simulink model "Mass_Springs_Systems"  (R2021b)
settings: Solver=ode4  StartTime=0.0  StopTime=30  FixedStep=.001  RelTol=1e-3  AbsTol=1e-3  EnableMultiTasking=on
model workspace (MAT data in the model file):
  cslide = 0.25
  iz = [0.192  0.091; 0.207  0.094; 0.221  0.104; 0.238  0.118; 0.251  0.141; 0.262  0.168; 0.268  0.205; 0.27  0.242; 0.267  0.277; 0.262  0.308; 0.246  0.348; 0.232  0.369; 0.206  0.39; 0.185  0.39; 0.16  0.377; 0.137  0.349; 0.126  0.325; 0.118  0.297; 0.114  0.265; 0.113  0.237; 0.118  0.191; 0.128  0.156; 0.139  0.13; 0.156  0.107; 0.175  0.096]
  m1 = 0
  m2 = 0
  m3 = 0
  one = [0.064  0.072; 0.088  0.03; 0.169  0.03; 0.168  0.458; 0.129  0.458; 0.128  0.073]
  smiData.RigidTransform.translation = [-21.5561986301 -14.8674859839 15.0728144895]
  smiData.RigidTransform.angle = 0
  smiData.RigidTransform.axis = [0 0 0]
  smiData.RigidTransform.ID = 'RootGround[rack-1]'
  smiData.Solid.mass = 0.0200061588425
  smiData.Solid.CoM = [0 0.838779102261 -0.00603396973069]
  smiData.Solid.MoI = [0.670200057653 0.669872690066 0.00366172739385]
  smiData.Solid.PoI = [5.56695055283e-05 0 0]
  smiData.Solid.color = [0.792156862745 0.819607843137 0.933333333333]
  smiData.Solid.opacity = 1
  smiData.Solid.ID = 'rack*:*Default'
  three = [0.252  0.12; 0.239  0.091; 0.214  0.068; 0.179  0.053; 0.14  0.052; 0.107  0.064; 0.083  0.082; 0.065  0.121; 0.075  0.155; 0.102  0.176; 0.129  0.188; 0.163  0.194; 0.182  0.194; 0.183  0.24; 0.131  0.247; 0.099  0.256; 0.068  0.28; 0.048  0.313; 0.047  0.345; 0.055  0.378; 0.084  0.41; 0.127  0.429; 0.179  0.43; 0.214  0.419; 0.246  0.396; 0.26  0.368; 0.269  0.344; 0.311  0.344; 0.303  0.374; 0.29  0.409; 0.262  0.442; 0.23  0.463; 0.18  0.475; 0.137  0.476; 0.097  0.465; 0.057  0.441; 0.028  0.411; 0.011  0.374; 0.006  0.353; 0.01  0.295; 0.028  0.258; 0.05  0.233; 0.08  0.214; 0.06  0.196; 0.041  0.175; 0.029  0.135; 0.029  0.104; 0.043  0.066; 0.074  0.032; 0.106  0.015; 0.147  0.006; 0.187  0.007; 0.223  0.021; 0.255  0.044; 0.278  0.081; 0.294  0.119]
  two = [0.081  0.154; 0.042  0.154; 0.05  0.108; 0.06  0.085; 0.082  0.055; 0.106  0.033; 0.135  0.02; 0.161  0.013; 0.194  0.014; 0.226  0.02; 0.253  0.032; 0.279  0.054; 0.297  0.083; 0.305  0.109; 0.309  0.141; 0.306  0.168; 0.299  0.189; 0.281  0.221; 0.242  0.271; 0.119  0.401; 0.315  0.403; 0.314  0.445; 0.027  0.446; 0.242  0.214; 0.263  0.177; 0.272  0.145; 0.264  0.106; 0.243  0.079; 0.208  0.059; 0.185  0.058; 0.162  0.06; 0.133  0.067; 0.12  0.076; 0.102  0.092; 0.088  0.119; 0.085  0.134]
  xy_simple = [39.1661  19.7032018238; 3.8339  19.7032; -0.28263658  19.7032; -0.28263658  0; 43  0; 43  19.7032]
  zero = [0.2  0.026; 0.245  0.033; 0.288  0.063; 0.316  0.099; 0.335  0.149; 0.345  0.197; 0.347  0.246; 0.344  0.292; 0.338  0.339; 0.324  0.384; 0.3  0.429; 0.269  0.456; 0.223  0.475; 0.173  0.475; 0.132  0.46; 0.097  0.426; 0.072  0.383; 0.062  0.338; 0.058  0.289; 0.058  0.242; 0.059  0.192; 0.068  0.145; 0.083  0.102; 0.111  0.062; 0.149  0.037]
undefined symbols (not defined in the file): A, d1, d2, ha, X, Y, Z
libraries: sm_lib x6312, nesl_utility x38
(part 1 of 121)
settings Model: Creator=HP Owner  LastModifiedBy=acontr14
settings SolverCC: AutoScaleAbsTol=off  AlgebraicLoopSolver=TrustRegion
settings DataIOCC: MaxDataPoints=10000
settings OptimizationCC: LifeSpan=inf
settings DebuggingCC: AllowSymbolicDim=off  SFUnexpectedBacktrackingDiag=warning  SFNoUnconditionalDefaultTransitionDiag=warning  SFExecutionAtInitializationDiag=none  SFMachineParentedDataDiag=warning  ArithmeticOperatorsInVariantConditions=warning
settings SFSimCC: SimUseLocalCustomCode=off  CustomCodeUndefinedFunction=UseInterfaceOnly
settings RTWCC: RTWUseLocalCustomCode=off
settings CodeAppCC: StateflowObjectComments=on
settings GRTTargetCC: TargetLangStandard=C89/C90 (ANSI)
settings ConfigComp: CovMetricSettings=dw  CovSaveCumulativeToWorkspaceVar=on  CovSaveSingleToWorkspaceVar=on  CovExternalEMLEnable=off  CovSFcnEnable=off
settings SimscapeCC: SimscapeLogType=all  SimscapeLogSimulationStatistics=on  SimscapeLogDataHistory=10000

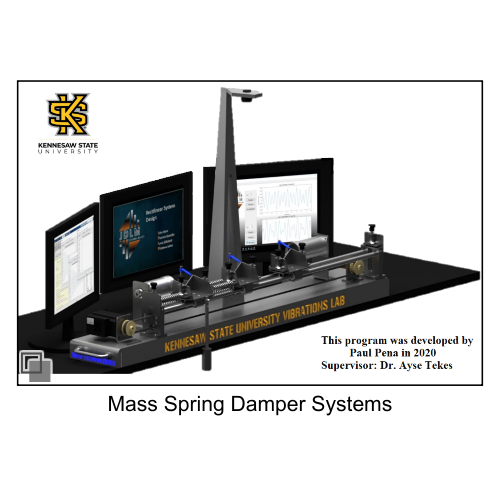
[thumbnail: Simulink's stored preview of the top-level diagram]
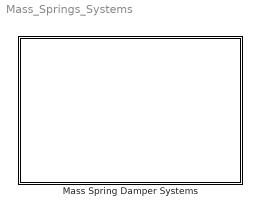
== system Mass_Springs_Systems ==
  Mass Spring Damper Systems : Subsystem  Variant=on  VariantControlMode=label  VariantControl=MS  LabelModeActiveChoice=22ms
      mask Display: image('$imagefile'); % Use "Edit Image" on toolstrip to change.

== system Mass_Springs_Systems/Mass Spring Damper Systems ==
  note: 1 Mass 1 Spring
  note: 3 Mass 3 Spring
  note: 2 Mass 2 Spring
  note: 1 Mass 2 Spring
  note: 2 Mass 3 Spring
  2Masses 2Springs : Subsystem  AncestorBlock=Lib/2Masses 2Springs  VariantControl=22ms  mask{m1=2, m2=1, k1=600, k2=400, d=1, s_f=.35, id1=2, id2=2, zero_forces=on, zerodis=off, force_type=Harmonic, Force=1, Har_Force=1, freq=sqrt(400/1.5)}
      mask prompts: m1 "Mass1 (kg)"; m2 "Mass2 (kg)"; k1 "K1 Spring Constant (N/m)"; k2 "K2 Spring Constant (N/m)"; d "Spring Damping (kg/s)"; s_f "Surface Friction (N/(m/s))"; id1 "M1 Initial Displacement (cm)"; id2 "M2 Initial Displacement (cm)"; zero_forces "Zero Forces"; zerodis "Zero Initial Displacement"; force_type "Force Response Type"; Force "Magnitude(N)"; Har_Force "Magnitude(N)"; freq "Frequency(rad/s)"
      mask init:
      | switch force_type
      |     case 1
      |         Har_Force = 0;
      |         freq = 0;
      |     case 2
      |         Force = 0;
      | end
      | if zero_forces == 1
      |     Har_Force = 0;
      |     Force = 0;
      |     freq = 0;
      | end
      | 
      | if zerodis == 1
      |     id1=0;
      |     id2=0;
      | end
      mask Callback zero_forces:
      | % Enable and disable parameters
      | 
      | % Get the value of the Enable Bias checkbox
      | % unchecked = 'off'
      | % checked = 'on'
      | enab = get_param(gcb,'zero_forces');
      | 
      | % Set the 'MaskEnables' property for each parameters
      | if strcmp(enab,'on')
      |     set_param(gcb,'MaskVisibilities',{'on','on','on','on','on','on','on','on','on','off','off','off','off','off'});
      | else
      |     set_param(gcb,'MaskVisibilities',{'on','on','on','on','on','on','on','on','on','on','on','on','on','on'});
      | end
      | 
      | % Note that the value of the bias is not handled here.
      | % See the Initialization tab
      mask Callback zerodis:
      | % Enable and disable parameters
      | 
      | % Get the value of the Enable Bias checkbox
      | % unchecked = 'off'
      | % checked = 'on'
      | enab = get_param(gcb,'zerodis');
      | 
      | % Set the 'MaskEnables' property for each parameters
      | if strcmp(enab,'on')
      |     set_param(gcb,'MaskEnables',{'on','on','on','on','on','on','off','off','on','on','on','on','on','on'});
      | else
      |     set_param(gcb,'MaskEnables',{'on','on','on','on','on','on','on','on','on','on','on','on','on','on'});
      | end
      | 
      | % Note that the value of the bias is not handled here.
      | % See the Initialization tab
      mask TypeOptions force_type: Step | Harmonic
      mask DialogControl Control4 Prompt: Update Model
      mask DialogControl Control4 Callback: set_param(bdroot,'SimulationCommand','update')
      mask DialogControl Control2 Prompt: Run Simulation
      mask DialogControl Control2 Callback: set_param(bdroot,'SimulationCommand','start')
      mask DialogControl Control3 Prompt: STOP Simulation
      mask DialogControl Control3 Callback: set_param(bdroot,'SimulationCommand','stop')
      mask DialogControl Control7 Prompt: Open Scope Plot
      mask DialogControl Control7 Callback: open(Simulink.BlockPath({'Mass_Springs_Systems/Mass Spring Damper Systems/2Masses 2Springs/Position'}))
      mask DialogControl Control14 Prompt: Frequency Plot
      mask DialogControl Control14 Callback:
      | cart1=evalin('base','out.pos1');
      | cart2=evalin('base','out.pos2');
      | time=evalin('base','out.tout');
      | 
      | Ts = time(2)-time(1);
      | fs = 1/Ts;
      | N = length(cart1);
      | 
      | Y1 = abs(fft(cart1)/N); % fft of cart1 data
      | Y1d = Y1(1:N/2+1); %single side spectrum
      | Y1d(2:end-1) = 2*Y1d(2:end-1); %amplitude adjustment
      | 
      | Y2 = abs(fft(cart2)/N);
      | Y2d = Y2(1:N/2+1);
      | Y2d(2:end-1) = 2*Y2d(2:end-1);
      | 
      | 
      | f = fs*(0:(N/2))/N; %create frequency vector
      | 
      | figure;
      | plot(f,Y1d); xlim([0 10]);
      | hold on;
      | plot(f,Y2d,'r')
      | hold off;
      mask DialogControl Control16 Prompt: Mode Ratios
      mask DialogControl Control16 Callback:
      | syms  w
      | m1=get_param(gcb,'m1');
      | m1=str2double(m1);
      | m2=get_param(gcb,'m2');
      | m2=str2double(m2);
      | k1=get_param(gcb,'k1');
      | k1=str2double(k1);
      | k2=get_param(gcb,'k2');
      | k2=str2double(k2);
      | M=[k1+k2-m1*w^2 -k2; -k2 k2-m2*w^2];
      | detM=det(M);
      | solution=double(solve(detM==0,w));
      | pos=solution>0;
      | wsolution=solution(pos);
      | w1=wsolution(1);
      | w2=wsolution(2);
      | f1=w1/(2*pi);
      | f2=w2/(2*pi);
      | M1=double(subs(M,w,w1));
      | Mode_Ratio_1=M1(1,1)/-M1(1,2);
      | M2=double(subs(M,w,w2));
      | Mode_Ratio_2=M2(1,1)/-M2(1,2);
      | %set_param(gcb,'MaskSelfModifiable','on');
      | % Get the mask object
      | mo = get_param(gcb,'MaskObject');
      | % Get the text object
      | tc = mo.getDialogControl('TextControl1');
      | % Change the string
      | tc.Prompt = string(Mode_Ratio_1);
      | % Get the text object
      | tc = mo.getDialogControl('TextControl2');
      | % Change the string
      | tc.Prompt = string(Mode_Ratio_2);
      mask DialogControl Container6 Prompt: Variables
      mask DialogControl Control13 Prompt: (Add text here)
      mask DialogControl Container8 Prompt: Free Response
      mask DialogControl Container11 Prompt: Free Response
      mask DialogControl Control17 Prompt: Mode Ratio of Mass 1:
      mask DialogControl TextControl1 Prompt: 1.6861
      mask DialogControl Control19 Prompt: Mode Ratio of Mass 2:
      mask DialogControl TextControl2 Prompt: -1.1861
      mask DialogControl Control10 Prompt: "Check Box below for Only Free Response"
      mask DialogControl Container19 Prompt: Forced Response
      mask DialogControl Container10 Prompt: Forced Response
      mask DialogControl Control9 Prompt: Uncheck "Zero Forces" in Free Response Tab to add Forced Response
      mask DialogControl Container13 Prompt: Step Response
      mask DialogControl Container16 Prompt: Harmonic Response
      mask Display: image('$imagefile'); % Use "Edit Image" on toolstrip to change.
  2Masses 3Springs : Subsystem  AncestorBlock=Lib/2Masses 3Springs  VariantControl=23ms  mask{m1=2, m2=2, k1=700, k2=300, k3=700, d=1/3, s_f=0, id1=3.500, id2=-3.500, zero_forces=on, zerodis=off, force_type=Harmonic, Force=5, Har_Force=3, freq=20}
      mask prompts: m1 "Mass1 (kg)"; m2 "Mass2 (kg)"; k1 "K1 Spring Constant (N/m)"; k2 "K2 Spring Constant (N/m)"; k3 "K3 Spring Constant (N/m)"; d "Spring Damping (kg/s)"; s_f "Surface Friction (N/(m/s))"; id1 "M1 Initial Displacement (cm)"; id2 "M2 Initial Displacement (cm)"; zero_forces "Zero Forces"; zerodis "Zero Initial Displacement"; force_type "Force Response Type"; Force "Magnitude(N)"; Har_Force "Magnitude(N)"; freq "Frequency(rad/s)"
      mask init:
      | switch force_type
      |     case 1
      |         Har_Force = 0;
      |         freq = 0;
      |     case 2
      |         Force = 0;
      | end
      | if zero_forces == 1
      |     Har_Force = 0;
      |     Force = 0;
      |     freq = 0;
      | end
      | 
      | if zerodis == 1
      |     id1 = 0;
      |     id2 = 0;
      | end
      mask Callback zero_forces:
      | % Enable and disable parameters
      | 
      | % Get the value of the Enable Bias checkbox
      | % unchecked = 'off'
      | % checked = 'on'
      | enab = get_param(gcb,'zero_forces');
      | 
      | % Set the 'MaskEnables' property for each parameters
      | if strcmp(enab,'on')
      |     set_param(gcb,'MaskVisibilities',{'on','on','on','on','on','on','on','on','on','on','off','off','off','off','off'});
      | else
      |     set_param(gcb,'MaskVisibilities',{'on','on','on','on','on','on','on','on','on','on','on','on','on','on','on'});
      | end
      | 
      | % Note that the value of the bias is not handled here.
      | % See the Initialization tab
      mask Callback zerodis:
      | % Enable and disable parameters
      | 
      | % Get the value of the Enable Bias checkbox
      | % unchecked = 'off'
      | % checked = 'on'
      | enab = get_param(gcb,'zerodis');
      | 
      | % Set the 'MaskEnables' property for each parameters
      | if strcmp(enab,'on')
      |     set_param(gcb,'MaskEnables',{'on','on','on','on','on','on','on','off','off','on','on','on','on','on','on'});
      | else
      |     set_param(gcb,'MaskEnables',{'on','on','on','on','on','on','on','on','on','on','on','on','on','on','on'});
      | end
      | 
      | % Note that the value of the bias is not handled here.
      | % See the Initialization tab
      mask TypeOptions force_type: Step | Harmonic
      mask DialogControl Control4 Prompt: Update Model
      mask DialogControl Control4 Callback: set_param(bdroot,'SimulationCommand','update')
      mask DialogControl Control14 Prompt: Run Simulation
      mask DialogControl Control14 Callback: set_param(bdroot,'SimulationCommand','start')
      mask DialogControl Control3 Prompt: STOP Simulation
      mask DialogControl Control3 Callback: set_param(bdroot,'SimulationCommand','stop')
      mask DialogControl Control7 Prompt: Open Scope Plot
      mask DialogControl Control7 Callback: open(Simulink.BlockPath({'Mass_Springs_Systems/Mass Spring Damper Systems/2Masses 3Springs/Position'}))
      mask DialogControl Control15 Prompt: Frequency Plot
      mask DialogControl Control15 Callback:
      | cart1=evalin('base','out.pos1');
      | cart2=evalin('base','out.pos2');
      | time=evalin('base','out.tout');
      | 
      | Ts = time(2)-time(1);
      | fs = 1/Ts;
      | N = length(cart1);
      | 
      | Y1 = abs(fft(cart1)/N); % fft of cart1 data
      | Y1d = Y1(1:N/2+1); %single side spectrum
      | Y1d(2:end-1) = 2*Y1d(2:end-1); %amplitude adjustment
      | 
      | Y2 = abs(fft(cart2)/N);
      | Y2d = Y2(1:N/2+1);
      | Y2d(2:end-1) = 2*Y2d(2:end-1);
      | 
      | 
      | f = fs*(0:(N/2))/N; %create frequency vector
      | 
      | figure;
      | plot(f,Y1d); xlim([0 10]);
      | hold on;
      | plot(f,Y2d,'r')
      mask DialogControl Control18 Prompt: Mode Ratios
      mask DialogControl Control18 Callback:
      | syms  w
      | m1=get_param(gcb,'m1');
      | m1=str2double(m1);
      | m2=get_param(gcb,'m2');
      | m2=str2double(m2);
      | k1=get_param(gcb,'k1');
      | k1=str2double(k1);
      | k2=get_param(gcb,'k2');
      | k2=str2double(k2);
      | k3=get_param(gcb,'k3');
      | k3=str2double(k3);
      | M=[k1+k2-m1*w^2 -k2; -k2 k2+k3-m2*w^2];
      | detM=det(M);
      | solution=double(solve(detM==0,w));
      | pos=solution>0;
      | wsolution=solution(pos);
      | w1=wsolution(1);
      | w2=wsolution(2);
      | f1=w1/(2*pi);
      | f2=w2/(2*pi);
      | M1=double(subs(M,w,w1)) ;
      | Mode_Ratio_1=M1(1,1)/-M1(1,2);
      | M2=double(subs(M,w,w2)) ;
      | Mode_Ratio_2=M2(1,1)/-M2(1,2);
      | %set_param(gcb,'MaskSelfModifiable','on');
      | % Get the mask object
      | mo = get_param(gcb,'MaskObject');
      | % Get the text object
      | tc = mo.getDialogControl('TextControl1');
      | % Change the string
      | tc.Prompt = string(Mode_Ratio_1);
      | % Get the text object
      | tc = mo.getDialogControl('TextControl2');
      | % Change the string
      | tc.Prompt = string(Mode_Ratio_2);
      mask DialogControl Container6 Prompt: Variables
      mask DialogControl Container8 Prompt: Free Response
      mask DialogControl Container11 Prompt: Free Response
      mask DialogControl Control21 Prompt: Mode Ratio of Mass1:
      mask DialogControl TextControl1 Prompt: 1
      mask DialogControl Control22 Prompt: Mode Ratio of Mass 2:
      mask DialogControl TextControl2 Prompt: -1
      mask DialogControl Control10 Prompt: "Check Box below for Only Free Response"
      mask DialogControl Container19 Prompt: Forced Response
      mask DialogControl Container10 Prompt: Forced Response
      mask DialogControl Control9 Prompt: Uncheck "Zero Forces" in Free Response Tab to add Forced Response
      mask DialogControl Container13 Prompt: Step Response
      mask DialogControl Container16 Prompt: Harmonic Response
      mask Display: image('$imagefile'); % Use "Edit Image" on toolstrip to change.
  3Masses 3Springs : Subsystem  AncestorBlock=Lib/3Masses 3Springs  VariantControl=33ms  mask{m1=1, m2=1, m3=1, k1=100, k2=100, k3=100, d=1, s_f=0, d1=3.500, d2=3.500, d3=3.500, zero_forces=off, zerodis=off, force_type=Step, Force=5, Har_Force=6, freq=20}
      mask prompts: m1 "Mass1 (kg)"; m2 "Mass2 (kg)"; m3 "Mass3 (kg)"; k1 "K1 Spring Constant (N/m)"; k2 "K2 Spring Constant (N/m)"; k3 "K3 Spring Constant (N/m)"; d "Spring Damping (kg/s)"; s_f "Surface Friction (N/(m/s))"; d1 "M1 Initial Displacement (cm)"; d2 "M2 Initial Displacement (cm)"; d3 "M3 Initial Displacement (cm)"; zero_forces "Zero Forces"; zerodis "Zero Initial Displacement"; force_type "Force Response Type"; Force "Magnitude(N)"; Har_Force "Magnitude(N)"; freq "Frequency(rad/s)"
      mask init:
      | switch force_type
      |     case 1
      |         Har_Force = 0;
      |         freq = 0;
      |     case 2
      |         Force = 0;
      | end
      | if zero_forces == 1
      |     Har_Force = 0;
      |     Force = 0;
      |     freq = 0;
      | end
      | 
      | if zerodis == 1
      |     id1 = 0;
      |     id2 = 0;
      |     id3 = 0;
      | end
      mask Callback zero_forces:
      | % Enable and disable parameters
      | 
      | % Get the value of the Enable Bias checkbox
      | % unchecked = 'off'
      | % checked = 'on'
      | enab = get_param(gcb,'zero_forces');
      | 
      | % Set the 'MaskEnables' property for each parameters
      | if strcmp(enab,'on')
      |     set_param(gcb,'MaskVisibilities',{'on','on','on','on','on','on','on','on','on','on','on','on','off','off','off','off','off'});
      | else
      |     set_param(gcb,'MaskVisibilities',{'on','on','on','on','on','on','on','on','on','on','on','on','on','on','on','on','on'});
      | end
      | 
      | % Note that the value of the bias is not handled here.
      | % See the Initialization tab
      mask Callback zerodis:
      | % Enable and disable parameters
      | 
      | % Get the value of the Enable Bias checkbox
      | % unchecked = 'off'
      | % checked = 'on'
      | enab = get_param(gcb,'zerodis');
      | 
      | % Set the 'MaskEnables' property for each parameters
      | if strcmp(enab,'on')
      |     set_param(gcb,'MaskEnables',{'on','on','on','on','on','on','on','on','off','off','off','on','on','on','on','on','on'});
      | else
      |     set_param(gcb,'MaskEnables',{'on','on','on','on','on','on','on','on','on','on','on','on','on','on','on','on','on'});
      | end
      | 
      | % Note that the value of the bias is not handled here.
      | % See the Initialization tab
      mask TypeOptions force_type: Step | Harmonic
      mask DialogControl Control4 Prompt: Update Model
      mask DialogControl Control4 Callback: set_param(bdroot,'SimulationCommand','update')
      mask DialogControl Control2 Prompt: Run Simulation
      mask DialogControl Control2 Callback: set_param(bdroot,'SimulationCommand','start')
      mask DialogControl Control3 Prompt: STOP Simulation
      mask DialogControl Control3 Callback: set_param(bdroot,'SimulationCommand','stop')
      mask DialogControl Control7 Prompt: Open Scope Plot
      mask DialogControl Control7 Callback: open(Simulink.BlockPath({'Mass_Springs_Systems/Mass Spring Damper Systems/3Masses 3Springs/Position'}))
      mask DialogControl Control14 Prompt: Frequency Plot
      mask DialogControl Control14 Callback:
      | cart1=evalin('base','out.pos1');
      | cart2=evalin('base','out.pos2');
      | cart3=evalin('base','out.pos3');
      | time=evalin('base','out.tout');
      | 
      | Ts = time(2)-time(1);
      | fs = 1/Ts;
      | N = length(cart1);
      | 
      | Y1 = abs(fft(cart1)/N); % fft of cart1 data
      | Y1d = Y1(1:N/2+1); %single side spectrum
      | Y1d(2:end-1) = 2*Y1d(2:end-1); %amplitude adjustment
      | 
      | Y2 = abs(fft(cart2)/N);
      | Y2d = Y2(1:N/2+1);
      | Y2d(2:end-1) = 2*Y2d(2:end-1);
      | 
      | Y3 = abs(fft(cart3)/N);
      | Y3d = Y3(1:N/2+1);
      | Y3d(2:end-1) = 2*Y3d(2:end-1);
      | 
      | f = fs*(0:(N/2))/N; %create frequency vector
      | 
      | figure;
      | plot(f,Y1d); xlim([0 10]);
      | hold on;
      | plot(f,Y2d,'r')
      | plot(f,Y3d,'g')
      mask DialogControl Container6 Prompt: Variables
      mask DialogControl Container8 Prompt: Free Response
      mask DialogControl Container11 Prompt: Free Response
      mask DialogControl Control10 Prompt: "Check Box below for Only Free Response"
      mask DialogControl Container19 Prompt: Forced Response
      mask DialogControl Container10 Prompt: Forced Response
      mask DialogControl Control9 Prompt: Uncheck "Zero Forces" in Free Response Tab to add Forced Response
      mask DialogControl Container13 Prompt: Step Response
      mask DialogControl Container16 Prompt: Harmonic Response
      mask Display: image('$imagefile'); % Use "Edit Image" on toolstrip to change.
  Mass Spring : Subsystem  AncestorBlock=Lib/Mass Spring  VariantControl=11ms  mask{m1=2, k1=600, d1=1, s_f=.35, id1=-0.350, zero_forces=off, zerodis=on, force_type=Harmonic, Force=4, Har_Force=2, freq=sqrt(400/1.5)}
      mask prompts: m1 "Mass1 (kg)"; k1 "K1 Spring Constant (N/m)"; d1 "Spring Damping (kg/s)"; s_f "Surface Friction (N/(m/s))"; id1 "M1 Initial Displacement (cm)"; zero_forces "Zero Forces"; zerodis "Zero Initial Displacement"; force_type "Force Response Type"; Force "Magnitude(N)"; Har_Force "Magnitude(N)"; freq "Frequency(rad/s)"
      mask init:
      | switch force_type
      |     case 1
      |         Har_Force = 0;
      |         freq = 0;
      |     case 2
      |         Force = 0;
      | end
      | if zero_forces == 1
      |     Har_Force = 0;
      |     Force = 0;
      |     freq = 0;
      | end
      | 
      | if zerodis == 1
      |     id1 = 0;
      | end
      mask Callback zero_forces:
      | % Enable and disable parameters
      | 
      | % Get the value of the Enable Bias checkbox
      | % unchecked = 'off'
      | % checked = 'on'
      | enab = get_param(gcb,'zero_forces');
      | 
      | % Set the 'MaskEnables' property for each parameters
      | if strcmp(enab,'on')
      |     set_param(gcb,'MaskVisibilities',{'on','on','on','on','on','on','off','off','off','off','off'});
      | else
      |     set_param(gcb,'MaskVisibilities',{'on','on','on','on','on','on','on','on','on','on','on'});
      | end
      | 
      | % Note that the value of the bias is not handled here.
      | % See the Initialization tab
      mask Callback zerodis:
      | % Enable and disable parameters
      | 
      | % Get the value of the Enable Bias checkbox
      | % unchecked = 'off'
      | % checked = 'on'
      | enab = get_param(gcb,'zerodis');
      | 
      | % Set the 'MaskEnables' property for each parameters
      | if strcmp(enab,'on')
      |     set_param(gcb,'MaskEnables',{'on','on','on','on','off','on','on','on','on','on','on'});
      | else
      |     set_param(gcb,'MaskEnables',{'on','on','on','on','on','on','on','on','on','on','on'});
      | end
      | 
      | % Note that the value of the bias is not handled here.
      | % See the Initialization tab
      mask TypeOptions force_type: Step | Harmonic
      mask DialogControl Control4 Prompt: Update Model
      mask DialogControl Control4 Callback: set_param(bdroot,'SimulationCommand','update')
      mask DialogControl Control2 Prompt: Run Simulation
      mask DialogControl Control2 Callback: set_param(bdroot,'SimulationCommand','start')
      mask DialogControl Control3 Prompt: STOP Simulation
      mask DialogControl Control3 Callback: set_param(bdroot,'SimulationCommand','stop')
      mask DialogControl Control7 Prompt: Open Scope Plot
      mask DialogControl Control7 Callback: open(Simulink.BlockPath({'Mass_Springs_Systems/Mass Spring Damper Systems/Mass Spring/Position'}))
      mask DialogControl Container6 Prompt: Variables
      mask DialogControl Container8 Prompt: Free Response
      mask DialogControl Container11 Prompt: Free Response
      mask DialogControl Control10 Prompt: "Check Box below for Only Free Response"
      mask DialogControl Container19 Prompt: Forced Response
      mask DialogControl Container10 Prompt: Forced Response
      mask DialogControl Control9 Prompt: Uncheck "Zero Forces" in Free Response Tab to add Forced Response
      mask DialogControl Container13 Prompt: Step Response
      mask DialogControl Container16 Prompt: Harmonic Response
      mask Display: image('$imagefile'); % Use "Edit Image" on toolstrip to change.
  Spring Mass Spring : Subsystem  AncestorBlock=Lib/Spring Mass Spring  VariantControl=12ms  mask{m1=3, k1=200, k2=600, d=1, s_f=0, id1=1, zero_forces=on, zerodis=off, force_type=Harmonic, Force=3, Har_Force=3, freq=1}
      mask prompts: m1 "Mass1 (kg)"; k1 "K1 Spring Constant (N/m)"; k2 "K2 Spring Constant (N/m)"; d "Spring Damping (kg/s)"; s_f "Surface Friction (N/(m/s))"; id1 "M1 Initial Displacement (cm)"; zero_forces "Zero Forces"; zerodis "Zero Initial Displacement"; force_type "Force Response Type"; Force "Magnitude(N)"; Har_Force "Magnitude(N)"; freq "Frequency(rad/s)"
      mask init:
      | switch force_type
      |     case 1
      |         Har_Force = 0;
      |         freq = 0;
      |     case 2
      |         Force = 0;
      | end
      | if zero_forces == 1
      |     Har_Force = 0;
      |     Force = 0;
      |     freq = 0;
      | end
      | 
      | if zerodis == 1
      |     id1=0;
      | end
      mask Callback zero_forces:
      | % Enable and disable parameters
      | 
      | % Get the value of the Enable Bias checkbox
      | % unchecked = 'off'
      | % checked = 'on'
      | enab = get_param(gcb,'zero_forces');
      | 
      | % Set the 'MaskEnables' property for each parameters
      | if strcmp(enab,'on')
      |     set_param(gcb,'MaskVisibilities',{'on','on','on','on','on','on','on','off','off','off','off','off'});
      | else
      |     set_param(gcb,'MaskVisibilities',{'on','on','on','on','on','on','on','on','on','on','on','on'});
      | end
      | 
      | % Note that the value of the bias is not handled here.
      | % See the Initialization tab
      mask Callback zerodis:
      | % Enable and disable parameters
      | 
      | % Get the value of the Enable Bias checkbox
      | % unchecked = 'off'
      | % checked = 'on'
      | enab = get_param(gcb,'zerodis');
      | 
      | % Set the 'MaskEnables' property for each parameters
      | if strcmp(enab,'on')
      |     set_param(gcb,'MaskEnables',{'on','on','on','on','on','off','on','on','on','on','on','on'});
      | else
      |     set_param(gcb,'MaskEnables',{'on','on','on','on','on','on','on','on','on','on','on','on'});
      | end
      | 
      | % Note that the value of the bias is not handled here.
      | % See the Initialization tab
      mask TypeOptions force_type: Step | Harmonic
      mask DialogControl Control4 Prompt: Update Model
      mask DialogControl Control4 Callback: set_param(bdroot,'SimulationCommand','update')
      mask DialogControl Control2 Prompt: Run Simulation
      mask DialogControl Control2 Callback: set_param(bdroot,'SimulationCommand','start')
      mask DialogControl Control3 Prompt: STOP Simulation
      mask DialogControl Control3 Callback: set_param(bdroot,'SimulationCommand','stop')
      mask DialogControl Control7 Prompt: Open Scope Plot
      mask DialogControl Control7 Callback: open(Simulink.BlockPath({'Mass_Springs_Systems/Mass Spring Damper Systems/Spring Mass Spring/Position'}))
      mask DialogControl Container6 Prompt: Variables
      mask DialogControl Container8 Prompt: Free Response
      mask DialogControl Container11 Prompt: Free Response
      mask DialogControl Control10 Prompt: "Check Box below for Only Free Response"
      mask DialogControl Container19 Prompt: Forced Response
      mask DialogControl Container10 Prompt: Forced Response
      mask DialogControl Control9 Prompt: Uncheck "Zero Forces" in Free Response Tab to add Forced Response
      mask DialogControl Container13 Prompt: Step Response
      mask DialogControl Container16 Prompt: Harmonic Response
      mask Display: image('$imagefile'); % Use "Edit Image" on toolstrip to change.
